simulink model "BLDCmotorControl_FOC_R2017b_fixdt_speedDeriv"  (R2017b)
settings: Solver=FixedStepDiscrete  StartTime=0  StopTime=0.5  FixedStep=Ts  MaxStep=1e-6  RelTol=1e-6  AbsTol=1e-6  EnableMultiTasking=on
PreLoadFcn:
  | addpath(genpath('01_Libraries'));
  | addpath(genpath('02_Figures'));
InitFcn:
  | init_model;
values from neighbouring files (symbols this model uses):
  a_elecAngle = 60    [init_model_Ffwd.m]
  b_DCLinkCurrAvail = 0    [init_model_Ffwd.m]
  b_fieldWeakEna = 0    [init_model_Ffwd.m]
  b_selPhaABCurrMeas = 1    [init_model_Ffwd.m]
  cf_currFilt = 0.02    [init_model_Ffwd.m]
  cf_speedCoef = round(f_ctrl * a_mechAngle * (pi/180) * (30/pi))    [init_model_Ffwd.m]
  CTRL_COM = 0    [init_model_Ffwd.m]
  dV_openRate = 1000 * Ts_ctrl    (= 0.06)    [init_model_Ffwd.m]
  dz_cntTrnsDetHi = 40    [init_model_Ffwd.m]
  dz_cntTrnsDetLo = 20    [init_model_Ffwd.m]
  i_max = i_max * i_sca    (= 750)    [init_model_Ffwd.m]
  i_thresOutlier = 200    [init_model_Ffwd.m]
  id_fieldWeak_M1 = [  0   0  0.05  0.25    1    2    3    4  4.5  4.8   5   5] * i_sca    [init_model_Ffwd.m]
  id_Kb = 1000 * Ts_ctrl    (= 0.06)    [init_model_Ffwd.m]
  id_Ki = 80 * Ts_ctrl    (= 0.0048)    [init_model_Ffwd.m]
  id_Kp = 0.5    [init_model_Ffwd.m]
  iq_Kb = 1000 * Ts_ctrl    (= 0.06)    [init_model_Ffwd.m]
  iq_Ki = 100 * Ts_ctrl    (= 0.006)    [init_model_Ffwd.m]
  iq_Kp = 0.5    [init_model_Ffwd.m]
  iq_KpLimProt = 4    [init_model_Ffwd.m]
  n_commAcvLo = 15    [init_model_Ffwd.m]
  n_commDeacvHi = 30    [init_model_Ffwd.m]
  n_Kb = 1000 * Ts_ctrl    (= 0.06)    [init_model_Ffwd.m]
  n_Ki = 10 * Ts_ctrl    (= 0.0006)    [init_model_Ffwd.m]
  n_Kp = 1    [init_model_Ffwd.m]
  n_KpLimProt = 5    [init_model_Ffwd.m]
  n_max = 800    [init_model_Ffwd.m]
  n_stdStillDet = 3    [init_model_Ffwd.m]
  OPEN_MODE = 0    [init_model_Ffwd.m]
  r_cos_M1 = cos((a_elecAngle_XA + 30)*(pi/180))    [init_model_Ffwd.m]
  r_sin_M1 = sin((a_elecAngle_XA + 30)*(pi/180))    [init_model_Ffwd.m]
  r_whl = 6.5 * 2.54 * 1e-2 / 2    (= 0.08255)    [init_model_Ffwd.m]
  SPD_MODE = 2    [init_model_Ffwd.m]
  TRQ_MODE = 3    [init_model_Ffwd.m]
  Ts = 5e-6    (= 5e-06)    [init_model_Ffwd.m]    (also in pe_electric_engine_dyno_data.m = 1e-05)
  Ts_ctrl = 6e-5    (= 6e-05)    [init_model_Ffwd.m]
  vec_hallToPos = [0 2 0 1 4 3 5 0]    [init_model_Ffwd.m]
  VLT_MODE = 1    [init_model_Ffwd.m]
  z_commutMap_M1 = [-1 -1  0  1  1  0 ... (first row only)    [init_model_Ffwd.m]
  z_ctrlModReq = 1    [init_model_Ffwd.m]
  z_ctrlTypSel = 1    [init_model_Ffwd.m]
  z_maxCntRst = 2000    [init_model_Ffwd.m]
undefined symbols (not defined in the file or in its folder): DiscIntNeverNeededParam, i_qMax_M1, sigbuilder_block, V_dMax, V_max, V_min, V_qMax_M1
libraries: simulink x11, BLDC_controller_Lib x9, powerlib x6, simulink_extras x1, pePwmGenerator x1
(part 2 of 3)

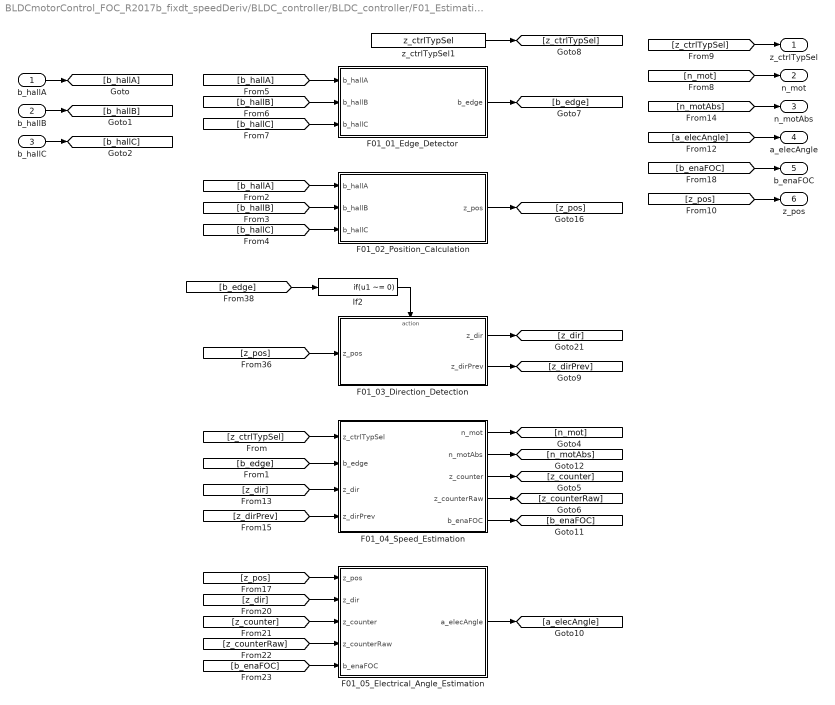
== system BLDCmotorControl_FOC_R2017b_fixdt_speedDeriv/BLDC_controller/BLDC_controller/F01_Estimations ==
  b_hallA : Inport
  b_hallB : Inport  Port=2
  b_hallC : Inport  Port=3
  F01_01_Edge_Detector : Subsystem
  F01_02_Position_Calculation : Subsystem
  F01_03_Direction_Detection : Subsystem
  F01_04_Speed_Estimation : Subsystem
  F01_05_Electrical_Angle_Estimation : Subsystem
  If2 : If  IfExpression=u1 ~= 0  ShowElse=off
  z_ctrlTypSel1 : Constant  Value=z_ctrlTypSel  OutDataTypeStr=uint8
  z_ctrlTypSel : Outport  OutputWhenDisabled=reset  InitialOutput=0
  "n_mot " : Outport  Port=2  OutputWhenDisabled=reset  InitialOutput=0
  n_motAbs : Outport  Port=3  OutputWhenDisabled=reset  InitialOutput=0
  a_elecAngle : Outport  Port=4  OutputWhenDisabled=reset  InitialOutput=0
  b_enaFOC : Outport  Port=5
  z_pos : Outport  Port=6  OutputWhenDisabled=reset  InitialOutput=0
  wires:
  If2/1 -> F01_03_Direction_Detection/Action
  [b_edge] -> If2/1
  [z_pos] -> F01_03_Direction_Detection/1(z_pos)
  [b_hallA] -> F01_01_Edge_Detector/1(b_hallA)
  F01_01_Edge_Detector/1("b_edge ") -> [b_edge]
  F01_03_Direction_Detection/1(z_dir) -> [z_dir]
  [b_hallB] -> F01_01_Edge_Detector/2(b_hallB)
  [b_hallC] -> F01_01_Edge_Detector/3(b_hallC)
  b_hallA/1 -> [b_hallA]
  b_hallB/1 -> [b_hallB]
  b_hallC/1 -> [b_hallC]
  [b_hallC] -> F01_02_Position_Calculation/3(b_hallC)
  [b_hallB] -> F01_02_Position_Calculation/2(b_hallB)
  [b_hallA] -> F01_02_Position_Calculation/1(b_hallA)
  F01_02_Position_Calculation/1("z_pos ") -> [z_pos]
  [b_edge] -> F01_04_Speed_Estimation/2(b_edge)
  F01_04_Speed_Estimation/1(n_mot) -> [n_mot]
  [n_mot] -> "n_mot "/1
  [z_pos] -> z_pos/1
  [z_dir] -> F01_04_Speed_Estimation/3(z_dir)
  F01_04_Speed_Estimation/3(z_counter) -> [z_counter]
  F01_04_Speed_Estimation/4(z_counterRaw) -> [z_counterRaw]
  F01_03_Direction_Detection/2(z_dirPrev) -> [z_dirPrev]
  [z_dirPrev] -> F01_04_Speed_Estimation/4(z_dirPrev)
  [z_pos] -> F01_05_Electrical_Angle_Estimation/1(z_pos)
  [z_dir] -> F01_05_Electrical_Angle_Estimation/2(z_dir)
  [z_counter] -> F01_05_Electrical_Angle_Estimation/3(z_counter)
  [z_counterRaw] -> F01_05_Electrical_Angle_Estimation/4(z_counterRaw)
  [b_enaFOC] -> F01_05_Electrical_Angle_Estimation/5(b_enaFOC)
  z_ctrlTypSel1/1 -> [z_ctrlTypSel]
  F01_04_Speed_Estimation/5(b_enaFOC) -> [b_enaFOC]
  [z_ctrlTypSel] -> F01_04_Speed_Estimation/1(z_ctrlTypSel)
  [b_enaFOC] -> b_enaFOC/1
  [a_elecAngle] -> a_elecAngle/1
  F01_05_Electrical_Angle_Estimation/1(a_elecAngle) -> [a_elecAngle]
  F01_04_Speed_Estimation/2(n_motAbs) -> [n_motAbs]
  [n_motAbs] -> n_motAbs/1
  [z_ctrlTypSel] -> z_ctrlTypSel/1

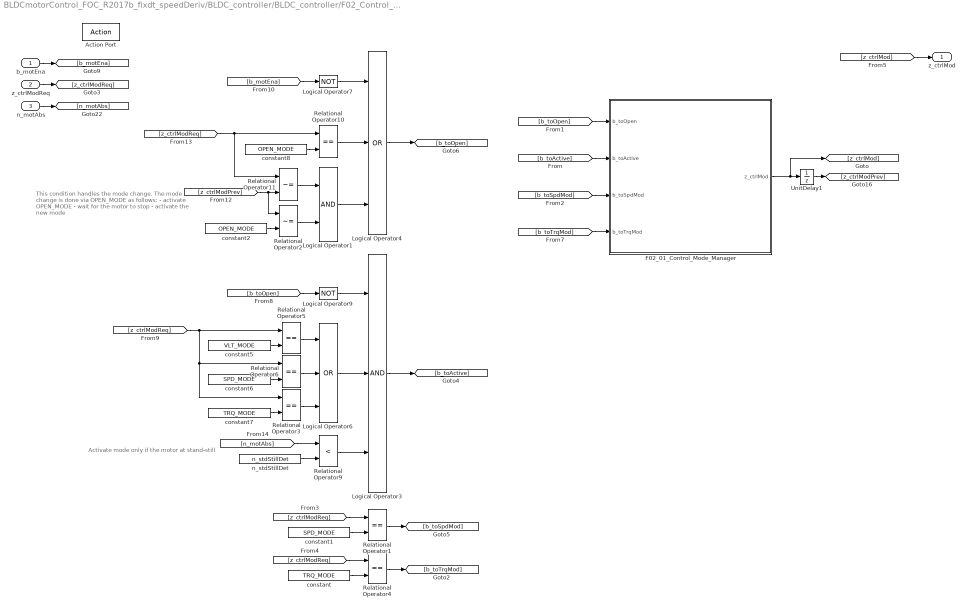
== system BLDCmotorControl_FOC_R2017b_fixdt_speedDeriv/BLDC_controller/BLDC_controller/F02_Control_Mode_Manager ==
  note: This condition handles the mode change. The mode change is done via OPEN_MODE as follows:
      | - activate OPEN_MODE
      | - wait for the motor to stop
      | - activate the new mode
  note: Activate mode only if the motor at stand-still
  b_motEna : Inport
  z_ctrlModReq : Inport  Port=2
  n_motAbs : Inport  Port=3
  Action Port : ActionPort  InitializeStates=reset  ActionType=then
  F02_01_Control_Mode_Manager : Stateflow chart  TreatAsAtomicUnit=on
  Logical Operator1 : Logic  AllPortsSameDT=off  OutDataTypeStr=boolean
  Logical Operator3 : Logic  Inputs=3  AllPortsSameDT=off  OutDataTypeStr=boolean
  Logical Operator4 : Logic  Operator=OR  Inputs=3  AllPortsSameDT=off  OutDataTypeStr=boolean
  Logical Operator6 : Logic  Operator=OR  Inputs=3  AllPortsSameDT=off  OutDataTypeStr=boolean
  Logical Operator7 : Logic  Operator=NOT  AllPortsSameDT=off  OutDataTypeStr=boolean
  Logical Operator9 : Logic  Operator=NOT  AllPortsSameDT=off  OutDataTypeStr=boolean
  Relational Operator{1,3..6,10} (6 alike) : RelationalOperator  Operator===  OutDataTypeStr=boolean  RndMeth=Simplest
  Relational Operator11 : RelationalOperator  Operator=~=  OutDataTypeStr=boolean  RndMeth=Simplest
  Relational Operator2 : RelationalOperator  Operator=~=  OutDataTypeStr=boolean  RndMeth=Simplest
  Relational Operator9 : RelationalOperator  Operator=<  OutDataTypeStr=boolean  RndMeth=Simplest
  UnitDelay1 : UnitDelay  SampleTime=-1
  constant : Constant  Value=TRQ_MODE  OutDataTypeStr=Inherit: Inherit via back propagation
  constant1 : Constant  Value=SPD_MODE  OutDataTypeStr=Inherit: Inherit via back propagation
  constant2 : Constant  Value=OPEN_MODE  OutDataTypeStr=Inherit: Inherit via back propagation
  constant5 : Constant  Value=VLT_MODE  OutDataTypeStr=Inherit: Inherit via back propagation
  constant6 : Constant  Value=SPD_MODE  OutDataTypeStr=Inherit: Inherit via back propagation
  constant7 : Constant  Value=TRQ_MODE  OutDataTypeStr=Inherit: Inherit via back propagation
  constant8 : Constant  Value=OPEN_MODE  OutDataTypeStr=Inherit: Inherit via back propagation
  n_stdStillDet : Constant  Value=n_stdStillDet  OutDataTypeStr=Inherit: Inherit via back propagation
  z_ctrlMod : Outport  OutputWhenDisabled=reset  InitialOutput=0
  wires:
  [z_ctrlMod] -> z_ctrlMod/1
  b_motEna/1 -> [b_motEna]
  [z_ctrlModReq] -> Relational Operator4/1
  constant/1 -> Relational Operator4/2
  Relational Operator4/1 -> [b_toTrqMod]
  [b_toOpen] -> F02_01_Control_Mode_Manager/1(b_toOpen)
  [b_toSpdMod] -> F02_01_Control_Mode_Manager/3(b_toSpdMod)
  z_ctrlModReq/1 -> [z_ctrlModReq]
  Relational Operator1/1 -> [b_toSpdMod]
  constant1/1 -> Relational Operator1/2
  [z_ctrlModReq] -> Relational Operator1/1
  [b_toTrqMod] -> F02_01_Control_Mode_Manager/4(b_toTrqMod)
  [z_ctrlModReq] -> Relational Operator6/1, Relational Operator3/1, Relational Operator5/1
  Relational Operator6/1 -> Logical Operator6/2
  constant6/1 -> Relational Operator6/2
  Relational Operator5/1 -> Logical Operator6/1
  constant5/1 -> Relational Operator5/2
  constant7/1 -> Relational Operator3/2
  Relational Operator3/1 -> Logical Operator6/3
  Logical Operator3/1 -> [b_toActive]
  [n_motAbs] -> Relational Operator9/1
  n_stdStillDet/1 -> Relational Operator9/2
  [z_ctrlModReq] -> Relational Operator11/1, Relational Operator10/1
  Logical Operator7/1 -> Logical Operator4/1
  [b_motEna] -> Logical Operator7/1
  Logical Operator4/1 -> [b_toOpen]
  [b_toOpen] -> Logical Operator9/1
  Logical Operator9/1 -> Logical Operator3/1
  UnitDelay1/1 -> [z_ctrlModPrev]
  F02_01_Control_Mode_Manager/1(z_ctrlMod) -> [z_ctrlMod], UnitDelay1/1
  [z_ctrlModPrev] -> Relational Operator2/1, Relational Operator11/2
  Relational Operator10/1 -> Logical Operator4/2
  constant8/1 -> Relational Operator10/2
  Logical Operator6/1 -> Logical Operator3/2
  Relational Operator9/1 -> Logical Operator3/3
  n_motAbs/1 -> [n_motAbs]
  [b_toActive] -> F02_01_Control_Mode_Manager/2(b_toActive)
  constant2/1 -> Relational Operator2/2
  Relational Operator11/1 -> Logical Operator1/1
  Relational Operator2/1 -> Logical Operator1/2
  Logical Operator1/1 -> Logical Operator4/3

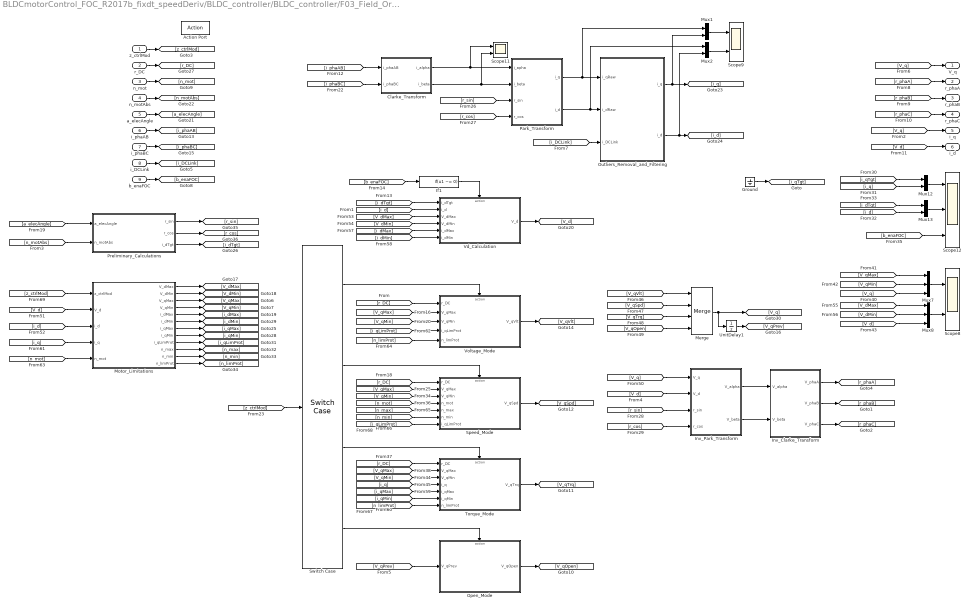
== system BLDCmotorControl_FOC_R2017b_fixdt_speedDeriv/BLDC_controller/BLDC_controller/F03_Field_Oriented_Control ==
  z_ctrlMod : Inport
  r_DC : Inport  Port=2
  n_mot : Inport  Port=3
  n_motAbs : Inport  Port=4
  a_elecAngle : Inport  Port=5
  i_phaAB : Inport  Port=6
  i_phaBC : Inport  Port=7
  i_DCLink : Inport  Port=8
  b_enaFOC : Inport  Port=9
  Action Port : ActionPort  InitializeStates=reset  ActionType=then
  Clarke_Transform : Subsystem
  Ground : Ground
  If1 : If  IfExpression=u1 ~= 0  ShowElse=off
  Inv_Clarke_Transform : Subsystem
  Inv_Park_Transform : Subsystem
  Merge : Merge  Inputs=4
  Motor_Limitations : Subsystem
  Mux{1..2,12..13} (4 alike) : Mux  Inputs=2
  Mux7 : Mux  Inputs=3
  Mux8 : Mux  Inputs=3
  Open_Mode : Subsystem
  Outliers_Removal_and_Filtering : Subsystem
  Park_Transform : Subsystem
  Preliminary_Calculations : Subsystem
  Scope11 : Scope  NumInputPorts=2
  Scope12 : Scope  NumInputPorts=3
  Scope8 : Scope  NumInputPorts=2
  Scope9 : Scope  NumInputPorts=2
  Speed_Mode : Subsystem
  Switch Case : SwitchCase  CaseConditions={VLT_MODE, SPD_MODE, TRQ_MODE}
  Torque_Mode : Subsystem
  UnitDelay1 : UnitDelay  SampleTime=-1
  Vd_Calculation : Subsystem
  Voltage_Mode : Subsystem
  V_q : Outport  OutputWhenDisabled=reset  InitialOutput=0
  r_phaA : Outport  Port=2  OutputWhenDisabled=reset  InitialOutput=0
  r_phaB : Outport  Port=3  OutputWhenDisabled=reset  InitialOutput=0
  "r_phaC " : Outport  Port=4  OutputWhenDisabled=reset  InitialOutput=0
  i_q : Outport  Port=5  OutputWhenDisabled=reset  InitialOutput=0
  i_d : Outport  Port=6  OutputWhenDisabled=reset  InitialOutput=0
  wires:
  [r_phaA] -> r_phaA/1
  [r_phaB] -> r_phaB/1
  [r_phaC] -> "r_phaC "/1
  Inv_Park_Transform/1(V_alpha) -> Inv_Clarke_Transform/1(V_alpha)
  Inv_Park_Transform/2(V_beta) -> Inv_Clarke_Transform/2(V_beta)
  i_phaAB/1 -> [i_phaAB]
  i_phaBC/1 -> [i_phaBC]
  Inv_Clarke_Transform/1(V_phaA) -> [r_phaA]
  Inv_Clarke_Transform/2(V_phaB) -> [r_phaB]
  Inv_Clarke_Transform/3(V_phaC) -> [r_phaC]
  Clarke_Transform/1(i_alpha) -> Scope11/1, Park_Transform/1(i_apha)
  Clarke_Transform/2(i_beta) -> Scope11/2, Park_Transform/2(i_beta)
  Mux12/1 -> Scope12/1
  Mux13/1 -> Scope12/2
  [r_sin] -> Park_Transform/3(r_sin)
  [r_cos] -> Park_Transform/4(r_cos)
  [r_sin] -> Inv_Park_Transform/3(r_sin)
  [r_cos] -> Inv_Park_Transform/4(r_cos)
  [i_qTgt] -> Mux12/1
  [i_q] -> Mux12/2
  [i_d] -> Mux13/2
  [i_dTgt] -> Mux13/1
  r_DC/1 -> [r_DC]
  [i_phaAB] -> Clarke_Transform/1(i_phaAB)
  [i_phaBC] -> Clarke_Transform/2(i_phaBC)
  [V_dMax] -> Mux8/1
  [V_d] -> Mux8/3
  Mux8/1 -> Scope8/2
  [V_dMin] -> Mux8/2
  [V_q] -> Mux7/3
  Mux7/1 -> Scope8/1
  [V_qMax] -> Mux7/1
  [V_qMin] -> Mux7/2
  [V_d] -> i_d/1
  [V_q] -> i_q/1
  [i_DCLink] -> Outliers_Removal_and_Filtering/3(i_DCLink)
  i_DCLink/1 -> [i_DCLink]
  Park_Transform/2(i_d) -> Mux2/1, Outliers_Removal_and_Filtering/2(i_dRaw)
  Park_Transform/1(i_q) -> Mux1/1, Outliers_Removal_and_Filtering/1(i_qRaw)
  Outliers_Removal_and_Filtering/1(i_q) -> Mux1/2, [i_q]
  Outliers_Removal_and_Filtering/2(i_d) -> Mux2/2, [i_d]
  [V_q] -> V_q/1
  Vd_Calculation/1(V_d) -> [V_d]
  [i_d] -> Vd_Calculation/2(i_d)
  [i_dTgt] -> Vd_Calculation/1(i_dTgt)
  b_enaFOC/1 -> [b_enaFOC]
  If1/1 -> Vd_Calculation/Action
  [b_enaFOC] -> If1/1
  [V_d] -> Inv_Park_Transform/2(V_d)
  z_ctrlMod/1 -> [z_ctrlMod]
  n_mot/1 -> [n_mot]
  [b_enaFOC] -> Scope12/3
  [z_ctrlMod] -> Switch Case/1
  [V_qPrev] -> Open_Mode/1(V_qPrev)
  Open_Mode/1(V_qOpen) -> [V_qOpen]
  Torque_Mode/1(V_qTrq) -> [V_qTrq]
  Speed_Mode/1(V_qSpd) -> [V_qSpd]
  Voltage_Mode/1(V_qVlt) -> [V_qVlt]
  [r_DC] -> Voltage_Mode/1(r_DC)
  [V_qMax] -> Voltage_Mode/2(V_qMax)
  [V_qMin] -> Voltage_Mode/3(V_qMin)
  [r_DC] -> Speed_Mode/1(r_DC)
  [V_qMax] -> Speed_Mode/2(V_qMax)
  [V_qMin] -> Speed_Mode/3(V_qMin)
  [n_mot] -> Speed_Mode/4(n_mot)
  [V_qMin] -> Torque_Mode/3(V_qMin)
  [V_qMax] -> Torque_Mode/2(V_qMax)
  [r_DC] -> Torque_Mode/1(r_DC)
  [i_q] -> Torque_Mode/4(i_q)
  Switch Case/1 -> Voltage_Mode/Action
  Switch Case/2 -> Speed_Mode/Action
  Switch Case/3 -> Torque_Mode/Action
  Switch Case/4 -> Open_Mode/Action
  [V_qVlt] -> Merge/1
  [V_qSpd] -> Merge/2
  [V_qTrq] -> Merge/3
  [V_qOpen] -> Merge/4
  [V_q] -> Inv_Park_Transform/1(V_q)
  Merge/1 -> UnitDelay1/1, [V_q]
  UnitDelay1/1 -> [V_qPrev]
  Motor_Limitations/3(V_qMax) -> [V_qMax]
  Motor_Limitations/4(V_qMin) -> [V_qMin]
  [V_d] -> Motor_Limitations/2(V_d)
  [i_d] -> Motor_Limitations/3(i_d)
  Motor_Limitations/2(V_dMin) -> [V_dMin]
  Motor_Limitations/1(V_dMax) -> [V_dMax]
  [V_dMax] -> Vd_Calculation/3(V_dMax)
  [V_dMin] -> Vd_Calculation/4(V_dMin)
  Motor_Limitations/5(i_dMax) -> [i_dMax]
  Motor_Limitations/6(i_dMin) -> [i_dMin]
  Motor_Limitations/7(i_qMax) -> [i_qMax]
  Motor_Limitations/8(i_qMin) -> [i_qMin]
  [i_dMax] -> Vd_Calculation/5(i_dMax)
  [i_dMin] -> Vd_Calculation/6(i_dMin)
  [i_qMax] -> Torque_Mode/5(i_qMax)
  [i_qMin] -> Torque_Mode/6(i_qMin)
  [i_q] -> Motor_Limitations/4(i_q)
  Motor_Limitations/9(i_qLimProt) -> [i_qLimProt]
  [i_qLimProt] -> Voltage_Mode/4(i_qLimProt)
  Motor_Limitations/11(n_min) -> [n_min]
  Motor_Limitations/10(n_max) -> [n_max]
  Motor_Limitations/12(n_limProt) -> [n_limProt]
  [n_mot] -> Motor_Limitations/5(n_mot)
  [n_limProt] -> Voltage_Mode/5(n_limProt)
  [n_max] -> Speed_Mode/5(n_max)
  [n_min] -> Speed_Mode/6(n_min)
  [n_limProt] -> Torque_Mode/7(n_limProt)
  [i_qLimProt] -> Speed_Mode/7(i_qLimProt)
  [z_ctrlMod] -> Motor_Limitations/1(z_ctrlMod)
  n_motAbs/1 -> [n_motAbs]
  Preliminary_Calculations/1(r_sin) -> [r_sin]
  Preliminary_Calculations/2(r_cos) -> [r_cos]
  [a_elecAngle] -> Preliminary_Calculations/1(a_elecAngle)
  Preliminary_Calculations/3(i_dTgt) -> [i_dTgt]
  [n_motAbs] -> Preliminary_Calculations/2(n_motAbs)
  a_elecAngle/1 -> [a_elecAngle]
  Ground/1 -> [i_qTgt]
  Mux1/1 -> Scope9/1
  Mux2/1 -> Scope9/2

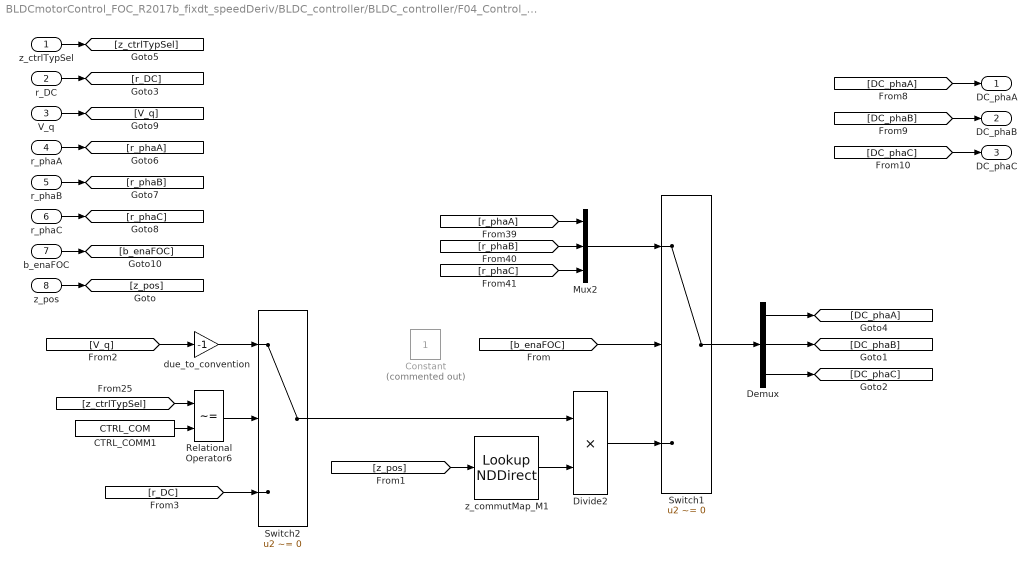
== system BLDCmotorControl_FOC_R2017b_fixdt_speedDeriv/BLDC_controller/BLDC_controller/F04_Control_Type_Management ==
  z_ctrlTypSel : Inport
  r_DC : Inport  Port=2
  V_q : Inport  Port=3
  r_phaA : Inport  Port=4
  r_phaB : Inport  Port=5
  r_phaC : Inport  Port=6
  b_enaFOC : Inport  Port=7
  z_pos : Inport  Port=8
  CTRL_COMM1 : Constant  Value=CTRL_COM  OutDataTypeStr=Inherit: Inherit via back propagation
  Constant : Constant  Commented=on  OutDataTypeStr=boolean
  Demux : Demux  Outputs=3
  Divide2 : Product  Inputs=**  RndMeth=Simplest  OutDataTypeStr=Inherit: Same as first input
  Mux2 : Mux  Inputs=3
  Relational Operator6 : RelationalOperator  Operator=~=  OutDataTypeStr=boolean  RndMeth=Simplest
  Switch1 : Switch  Criteria=u2 ~= 0  OutDataTypeStr=Inherit: Inherit via back propagation  RndMeth=Zero
  Switch2 : Switch  Criteria=u2 ~= 0  OutDataTypeStr=Inherit: Inherit via back propagation  RndMeth=Zero
  due_to_convention : Gain  Tag=struct('comment',struct('text','','placement',1),'logdata',struct('maxnumvals',inf,'plotchannels',[],'loggingmode',3,'channels',1),'output',struct('variable','','description','','name','$S_$B','width',1,'address','','max',NaN,'min',NaN,'class','default','type','CONTINUOUS','scaling','','lsb',1,'offset',0,'arb',0,'freeze',1,'unit','','autoscalingmode',1,'lowerheadroom',1,'upperheadroom',1,'headroomunit','bit','keepdatatype',1,'checkmin',0,'checkmax',0,'castoutput',0,'show',0),'gain',struct('variable','','description','','name','$S_$B_gain','width',1,'address','','max',NaN,'min',NaN,'class','default','type','CONTINUOUS','scaling','','lsb',1,'offset',0,'arb',0,'freeze',1,'unit','','keepdatatype',1,'value','1','scalar',0,'tolerance',1),'scalingvalid',0,'date',730486)  Gain=-1  RndMeth=Zero  SaturateOnIntegerOverflow=on  OutDataTypeStr=Inherit: Same as input  ParamDataTypeStr=Inherit: Same as input
  z_commutMap_M1 : LookupNDDirect  InputsSelectThisObjectFromTable=Column  Table=z_commutMap_M1  DiagnosticForOutOfRangeInput=None  TableDataTypeStr=int16
  DC_phaA : Outport  OutputWhenDisabled=reset  InitialOutput=0
  DC_phaB : Outport  Port=2  OutputWhenDisabled=reset  InitialOutput=0
  "DC_phaC " : Outport  Port=3  OutputWhenDisabled=reset  InitialOutput=0
  wires:
  Demux/3 -> [DC_phaC]
  Demux/2 -> [DC_phaB]
  Demux/1 -> [DC_phaA]
  z_pos/1 -> [z_pos]
  [DC_phaC] -> "DC_phaC "/1
  [DC_phaB] -> DC_phaB/1
  [DC_phaA] -> DC_phaA/1
  [z_pos] -> z_commutMap_M1/1
  Switch1/1 -> Demux/1
  r_phaA/1 -> [r_phaA]
  r_phaB/1 -> [r_phaB]
  r_phaC/1 -> [r_phaC]
  V_q/1 -> [V_q]
  [r_phaA] -> Mux2/1
  [r_phaB] -> Mux2/2
  [r_phaC] -> Mux2/3
  z_commutMap_M1/1 -> Divide2/2
  Divide2/1 -> Switch1/3
  b_enaFOC/1 -> [b_enaFOC]
  Mux2/1 -> Switch1/1
  [b_enaFOC] -> Switch1/2
  [V_q] -> due_to_convention/1
  Switch2/1 -> Divide2/1
  due_to_convention/1 -> Switch2/1
  [z_ctrlTypSel] -> Relational Operator6/1
  CTRL_COMM1/1 -> Relational Operator6/2
  Relational Operator6/1 -> Switch2/2
  r_DC/1 -> [r_DC]
  [r_DC] -> Switch2/3
  z_ctrlTypSel/1 -> [z_ctrlTypSel]

== system BLDCmotorControl_FOC_R2017b_fixdt_speedDeriv/BLDC_controller/BLDC_controller/Implemented_control_methods ==

== system BLDCmotorControl_FOC_R2017b_fixdt_speedDeriv/PWM_gates/PWM_generator1/__InputSSForSFun__ ==
  DC : Inport  SampleTime=Ts
  __UniqueOutportName__1__ : Outport
  wires:
  DC/1 -> __UniqueOutportName__1__/1

== system BLDCmotorControl_FOC_R2017b_fixdt_speedDeriv/PWM_gates/PWM_generator1/__OutputSSForSFun__ ==
  __UniqueInportName__1__ : Inport
  PWM : Outport
  wires:
  __UniqueInportName__1__/1 -> PWM/1

== system BLDCmotorControl_FOC_R2017b_fixdt_speedDeriv/PWM_gates/PWM_generator12/__InputSSForSFun__ ==
  DC : Inport  SampleTime=Ts
  __UniqueOutportName__1__ : Outport
  wires:
  DC/1 -> __UniqueOutportName__1__/1

== system BLDCmotorControl_FOC_R2017b_fixdt_speedDeriv/PWM_gates/PWM_generator12/__OutputSSForSFun__ ==
  __UniqueInportName__1__ : Inport
  PWM : Outport
  wires:
  __UniqueInportName__1__/1 -> PWM/1

== system BLDCmotorControl_FOC_R2017b_fixdt_speedDeriv/PWM_gates/PWM_generator2/__InputSSForSFun__ ==
  DC : Inport  SampleTime=Ts
  __UniqueOutportName__1__ : Outport
  wires:
  DC/1 -> __UniqueOutportName__1__/1

== system BLDCmotorControl_FOC_R2017b_fixdt_speedDeriv/PWM_gates/PWM_generator2/__OutputSSForSFun__ ==
  __UniqueInportName__1__ : Inport
  PWM : Outport
  wires:
  __UniqueInportName__1__/1 -> PWM/1

== system BLDCmotorControl_FOC_R2017b_fixdt_speedDeriv/PWM_gates/PWM_generator3/__InputSSForSFun__ ==
  DC : Inport  SampleTime=Ts
  __UniqueOutportName__1__ : Outport
  wires:
  DC/1 -> __UniqueOutportName__1__/1

== system BLDCmotorControl_FOC_R2017b_fixdt_speedDeriv/PWM_gates/PWM_generator3/__OutputSSForSFun__ ==
  __UniqueInportName__1__ : Inport
  PWM : Outport
  wires:
  __UniqueInportName__1__/1 -> PWM/1

== system BLDCmotorControl_FOC_R2017b_fixdt_speedDeriv/PWM_gates/PWM_generator4/__InputSSForSFun__ ==
  DC : Inport  SampleTime=Ts
  __UniqueOutportName__1__ : Outport
  wires:
  DC/1 -> __UniqueOutportName__1__/1

== system BLDCmotorControl_FOC_R2017b_fixdt_speedDeriv/PWM_gates/PWM_generator4/__OutputSSForSFun__ ==
  __UniqueInportName__1__ : Inport
  PWM : Outport
  wires:
  __UniqueInportName__1__/1 -> PWM/1

== system BLDCmotorControl_FOC_R2017b_fixdt_speedDeriv/PWM_gates/PWM_generator5/__InputSSForSFun__ ==
  DC : Inport  SampleTime=Ts
  __UniqueOutportName__1__ : Outport
  wires:
  DC/1 -> __UniqueOutportName__1__/1

== system BLDCmotorControl_FOC_R2017b_fixdt_speedDeriv/PWM_gates/PWM_generator5/__OutputSSForSFun__ ==
  __UniqueInportName__1__ : Inport
  PWM : Outport
  wires:
  __UniqueInportName__1__/1 -> PWM/1

== system BLDCmotorControl_FOC_R2017b_fixdt_speedDeriv/BLDC_controller/BLDC_controller/F01_Estimations/F01_01_Edge_Detector ==
  b_hallA : Inport
  b_hallB : Inport  Port=2
  b_hallC : Inport  Port=3
  Bitwise Operator : simulink/Logic and Bit Operations/Bitwise Operator  logicop=XOR  UseBitMask=off  NumInputPorts=6  BitMask=bin2dec('11011001')  BitMaskRealWorld=Stored Integer
  UnitDelay : UnitDelay  SampleTime=-1
  UnitDelay1 : UnitDelay  SampleTime=-1
  UnitDelay2 : UnitDelay  SampleTime=-1
  "b_edge " : Outport  OutputWhenDisabled=reset  InitialOutput=0
  wires:
  b_hallA/1 -> Bitwise Operator/1, UnitDelay/1
  b_hallC/1 -> Bitwise Operator/3, UnitDelay2/1
  b_hallB/1 -> Bitwise Operator/2, UnitDelay1/1
  Bitwise Operator/1 -> "b_edge "/1
  UnitDelay1/1 -> Bitwise Operator/5
  UnitDelay2/1 -> Bitwise Operator/6
  UnitDelay/1 -> Bitwise Operator/4

== system BLDCmotorControl_FOC_R2017b_fixdt_speedDeriv/BLDC_controller/BLDC_controller/F01_Estimations/F01_02_Position_Calculation ==
  note: This calculates the low resolution position based on Hall sensors.
  b_hallA : Inport
  b_hallB : Inport  Port=2
  b_hallC : Inport  Port=3
  Selector : Selector  IndexMode=Zero-based  InputPortWidth=length(vec_hallToPos)  IndexOptions=Index vector (port)  Indices=[1 3]  OutputSizes=1
  Sum : Sum  Inputs=+++  RndMeth=Simplest  OutDataTypeStr=Inherit: Same as first input
  g_Ha : Gain  Gain=4  OutDataTypeStr=Inherit: Inherit via back propagation  RndMeth=Zero  ParamDataTypeStr=Inherit: Same as input
  g_Hb : Gain  Gain=2  OutDataTypeStr=Inherit: Inherit via back propagation  RndMeth=Simplest  ParamDataTypeStr=Inherit: Same as input
  vec_hallToPos : Constant  Value=vec_hallToPos  OutDataTypeStr=int8
  "z_pos " : Outport  OutputWhenDisabled=reset  InitialOutput=0
  wires:
  b_hallC/1 -> Sum/3
  g_Ha/1 -> Sum/1
  g_Hb/1 -> Sum/2
  Sum/1 -> Selector/2
  b_hallA/1 -> g_Ha/1
  b_hallB/1 -> g_Hb/1
  vec_hallToPos/1 -> Selector/1
  Selector/1 -> "z_pos "/1

== system BLDCmotorControl_FOC_R2017b_fixdt_speedDeriv/BLDC_controller/BLDC_controller/F01_Estimations/F01_03_Direction_Detection ==
  z_pos : Inport
  Action Port : ActionPort  ActionType=then
  Constant20 : Constant  Value=-5  OutDataTypeStr=Inherit: Inherit via back propagation
  Constant23 : Constant  Value=-1  OutDataTypeStr=int8
  Constant24 : Constant  OutDataTypeStr=int8
  Constant8 : Constant  OutDataTypeStr=Inherit: Inherit via back propagation
  Logical Operator3 : Logic  Operator=OR  AllPortsSameDT=off  OutDataTypeStr=boolean
  Relational Operator1 : RelationalOperator  Operator===  OutDataTypeStr=boolean  RndMeth=Simplest
  Relational Operator6 : RelationalOperator  Operator===  OutDataTypeStr=boolean  RndMeth=Simplest
  Sum2 : Sum  Inputs=|+-  RndMeth=Zero  InputSameDT=on  OutDataTypeStr=Inherit: Same as first input
  Switch2 : Switch  Criteria=u2 ~= 0  OutDataTypeStr=Inherit: Inherit via back propagation  RndMeth=Simplest
  UnitDelay1 : UnitDelay  SampleTime=-1
  UnitDelay2 : UnitDelay  SampleTime=-1
  z_dir : Outport
  z_dirPrev : Outport  Port=2
  wires:
  UnitDelay2/1 -> Sum2/2
  Relational Operator1/1 -> Logical Operator3/1
  Constant8/1 -> Relational Operator1/2
  Sum2/1 -> Relational Operator6/1, Relational Operator1/1
  Relational Operator6/1 -> Logical Operator3/2
  Constant20/1 -> Relational Operator6/2
  Constant24/1 -> Switch2/1
  Constant23/1 -> Switch2/3
  Logical Operator3/1 -> Switch2/2
  z_pos/1 -> Sum2/1, UnitDelay2/1
  Switch2/1 -> UnitDelay1/1, z_dir/1
  UnitDelay1/1 -> z_dirPrev/1

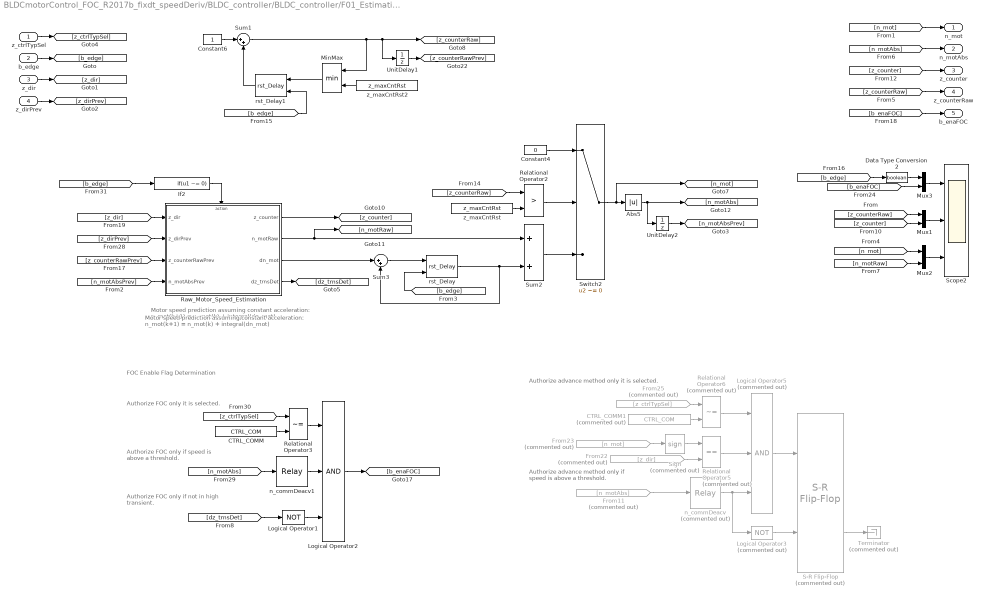
== system BLDCmotorControl_FOC_R2017b_fixdt_speedDeriv/BLDC_controller/BLDC_controller/F01_Estimations/F01_04_Speed_Estimation ==
  note: Motor speed prediction assuming constant acceleration:
      | n_mot(k+1) = n_mot(k) + integral(dn_mot)
  note: Authorize advance method only if speed is above a threshold.
  note: Authorize advance method only it is selected.
  note: FOC Enable Flag Determination
  note: Authorize FOC only if speed is above a threshold.
  note: Authorize FOC only if not in high transient.
  note: Authorize FOC only it is selected.
  note: Motor speed prediction assuming constant acceleration:
      | n_mot(k+1) = n_mot(k) + integral(dn_mot)
  z_ctrlTypSel : Inport
  b_edge : Inport  Port=2
  z_dir : Inport  Port=3
  z_dirPrev : Inport  Port=4
  Abs5 : Abs  OutDataTypeStr=Inherit: Inherit via back propagation  RndMeth=Zero
  CTRL_COMM : Constant  Value=CTRL_COM  OutDataTypeStr=Inherit: Inherit via back propagation
  CTRL_COMM1 : Constant  Commented=on  Value=CTRL_COM  OutDataTypeStr=Inherit: Inherit via back propagation
  Constant4 : Constant  Value=0  OutDataTypeStr=Inherit: Inherit via back propagation
  Constant6 : Constant  OutDataTypeStr=int16
  Data Type Conversion2 : DataTypeConversion  OutDataTypeStr=boolean
  From11 : From  Commented=on  GotoTag=n_motAbs
  From22 : From  Commented=on  GotoTag=z_dir
  From23 : From  Commented=on  GotoTag=n_mot
  From25 : From  Commented=on  GotoTag=z_ctrlTypSel
  If2 : If  IfExpression=u1 ~= 0  ShowElse=off
  Logical Operator1 : Logic  Operator=NOT  AllPortsSameDT=off  OutDataTypeStr=boolean
  Logical Operator2 : Logic  Inputs=3  AllPortsSameDT=off  OutDataTypeStr=boolean
  Logical Operator3 : Logic  Commented=on  Operator=NOT  AllPortsSameDT=off  OutDataTypeStr=boolean
  Logical Operator5 : Logic  Commented=on  Inputs=3  AllPortsSameDT=off  OutDataTypeStr=boolean
  MinMax : MinMax  Inputs=2
  Mux1 : Mux  Inputs=2
  Mux2 : Mux  Inputs=2
  Mux3 : Mux  Inputs=2
  Raw_Motor_Speed_Estimation : Subsystem
  Relational Operator2 : RelationalOperator  Operator=>  OutDataTypeStr=boolean  RndMeth=Simplest
  Relational Operator3 : RelationalOperator  Operator=~=  OutDataTypeStr=boolean  RndMeth=Simplest
  Relational Operator5 : RelationalOperator  Commented=on  Operator===  OutDataTypeStr=boolean  RndMeth=Simplest
  Relational Operator6 : RelationalOperator  Commented=on  Operator=~=  OutDataTypeStr=boolean  RndMeth=Simplest
  S-R Flip-Flop : simulink_extras/Flip Flops/S-R Flip-Flop  Commented=on  initial_condition=0
  Scope2 : Scope  NumInputPorts=3
  Sign : Signum  Commented=on
  Sum1 : Sum  Inputs=|++  RndMeth=Simplest  InputSameDT=on  OutDataTypeStr=Inherit: Same as first input
  Sum2 : Sum  RndMeth=Simplest  OutDataTypeStr=Inherit: Same as first input
  Sum3 : Sum  Inputs=|++  RndMeth=Simplest  OutDataTypeStr=Inherit: Same as first input
  Switch2 : Switch  Criteria=u2 ~= 0  OutDataTypeStr=Inherit: Inherit via back propagation  RndMeth=Zero
  Terminator : Terminator  Commented=on
  UnitDelay1 : UnitDelay  InitialCondition=z_maxCntRst  SampleTime=-1
  UnitDelay2 : UnitDelay  SampleTime=-1
  n_commDeacv : Relay  Commented=on  OnSwitchValue=n_commDeacvHi  OffSwitchValue=n_commAcvLo  OutDataTypeStr=boolean
  n_commDeacv1 : Relay  OnSwitchValue=n_commDeacvHi  OffSwitchValue=n_commAcvLo  OutDataTypeStr=boolean
  rst_Delay : BLDC_controller_Lib/rst_Delay  initVal=0
  rst_Delay1 : BLDC_controller_Lib/rst_Delay  initVal=z_maxCntRst
  z_maxCntRst : Constant  Value=z_maxCntRst  OutDataTypeStr=Inherit: Inherit via back propagation
  z_maxCntRst2 : Constant  Value=z_maxCntRst  OutDataTypeStr=Inherit: Inherit via back propagation
  n_mot : Outport
  n_motAbs : Outport  Port=2
  z_counter : Outport  Port=3  OutputWhenDisabled=reset  InitialOutput=0
  z_counterRaw : Outport  Port=4  OutputWhenDisabled=reset  InitialOutput=0
  b_enaFOC : Outport  Port=5
  wires:
  [n_motRaw] -> Mux2/2
  Mux2/1 -> Scope2/3
  [n_mot] -> Mux2/1
  Mux1/1 -> Scope2/2
  [z_counterRaw] -> Mux1/1
  [z_counter] -> Mux1/2
  [b_edge] -> Data Type Conversion2/1
  Constant6/1 -> Sum1/1
  Sum1/1 -> MinMax/1, [z_counterRaw], UnitDelay1/1
  b_edge/1 -> [b_edge]
  [n_mot] -> n_mot/1
  z_dir/1 -> [z_dir]
  [z_counter] -> z_counter/1
  [z_counterRaw] -> z_counterRaw/1
  UnitDelay1/1 -> [z_counterRawPrev]
  z_dirPrev/1 -> [z_dirPrev]
  Raw_Motor_Speed_Estimation/2(n_motRaw) -> Sum2/1, [n_motRaw]
  Raw_Motor_Speed_Estimation/3(dn_mot) -> Sum3/1
  [z_dir] -> Raw_Motor_Speed_Estimation/1(z_dir)
  Abs5/1 -> UnitDelay2/1, [n_motAbs]
  Raw_Motor_Speed_Estimation/1(z_counter) -> [z_counter]
  [z_dirPrev] -> Raw_Motor_Speed_Estimation/2(z_dirPrev)
  If2/1 -> Raw_Motor_Speed_Estimation/Action
  [z_counterRawPrev] -> Raw_Motor_Speed_Estimation/3(z_counterRawPrev)
  [b_enaFOC] -> b_enaFOC/1
  z_ctrlTypSel/1 -> [z_ctrlTypSel]
  rst_Delay/1 -> Sum2/2, Sum3/2
  [z_counterRaw] -> Relational Operator2/1
  z_maxCntRst/1 -> Relational Operator2/2
  Constant4/1 -> Switch2/1
  Sum2/1 -> Switch2/3
  Switch2/1 -> [n_mot], Abs5/1
  [b_edge] -> rst_Delay1/2
  z_maxCntRst2/1 -> MinMax/2
  rst_Delay1/1 -> Sum1/2
  MinMax/1 -> rst_Delay1/1
  S-R Flip-Flop/2 -> Terminator/1
  From11/1 -> n_commDeacv/1
  Logical Operator3/1 -> S-R Flip-Flop/2
  n_commDeacv/1 -> Logical Operator3/1, Logical Operator5/3
  Logical Operator5/1 -> S-R Flip-Flop/1
  Sign/1 -> Relational Operator5/1
  Relational Operator5/1 -> Logical Operator5/2
  Mux3/1 -> Scope2/1
  [b_enaFOC] -> Mux3/2
  Data Type Conversion2/1 -> Mux3/1
  From22/1 -> Relational Operator5/2
  From23/1 -> Sign/1
  From25/1 -> Relational Operator6/1
  CTRL_COMM1/1 -> Relational Operator6/2
  Relational Operator6/1 -> Logical Operator5/1
  [b_edge] -> If2/1
  Relational Operator2/1 -> Switch2/2
  UnitDelay2/1 -> [n_motAbsPrev]
  [n_motAbsPrev] -> Raw_Motor_Speed_Estimation/4(n_motAbsPrev)
  Sum3/1 -> rst_Delay/1
  [b_edge] -> rst_Delay/2
  [n_motAbs] -> n_motAbs/1
  CTRL_COMM/1 -> Relational Operator3/2
  [z_ctrlTypSel] -> Relational Operator3/1
  [n_motAbs] -> n_commDeacv1/1
  Raw_Motor_Speed_Estimation/4(dz_trnsDet) -> [dz_trnsDet]
  Relational Operator3/1 -> Logical Operator2/1
  n_commDeacv1/1 -> Logical Operator2/2
  Logical Operator1/1 -> Logical Operator2/3
  Logical Operator2/1 -> [b_enaFOC]
  [dz_trnsDet] -> Logical Operator1/1

== system BLDCmotorControl_FOC_R2017b_fixdt_speedDeriv/BLDC_controller/BLDC_controller/F01_Estimations/F01_05_Electrical_Angle_Estimation ==
  note: Electrical angle calculation
  note: This switch is to manage the situation when FOC control method is not enabled.
  z_pos : Inport
  z_dir : Inport  Port=2
  z_counter : Inport  Port=3
  z_counterRaw : Inport  Port=4
  b_enaFOC : Inport  Port=5
  Constant16 : Constant  OutDataTypeStr=Inherit: Inherit via back propagation
  Constant2 : Constant  OutDataTypeStr=Inherit: Inherit via back propagation
  Divide4 : Product  Inputs=*/*  RndMeth=Simplest  SaturateOnIntegerOverflow=on  OutDataTypeStr=Inherit: Same as first input
  Divide5 : Product  Inputs=**  RndMeth=Simplest  OutDataTypeStr=Inherit: Same as first input
  Mux : Mux  Inputs=2
  Product6 : Product  OutDataTypeStr=Inherit: Inherit via back propagation  RndMeth=Simplest
  Relational Operator7 : RelationalOperator  Operator===  OutDataTypeStr=boolean  RndMeth=Simplest
  Scope : Scope  NumInputPorts=2
  Sum1 : Sum  RndMeth=Simplest  OutDataTypeStr=Inherit: Same as first input
  Sum2 : Sum  RndMeth=Simplest  OutDataTypeStr=Inherit: Same as first input
  Switch1 : Switch  Criteria=u2 ~= 0  OutDataTypeStr=Inherit: Inherit via back propagation  RndMeth=Zero
  Switch3 : Switch  Criteria=u2 ~= 0  OutDataTypeStr=Inherit: Inherit via back propagation  RndMeth=Zero
  a_elecAngle1 : Constant  Value=a_elecAngle  OutDataTypeStr=fixdt(1,16,6)
  a_elecAngle : Outport  OutputWhenDisabled=reset  InitialOutput=0
  wires:
  z_pos/1 -> [z_pos]
  z_dir/1 -> [z_dir]
  Mux/1 -> Scope/1
  [a_elecAngle] -> Mux/1
  [a_elecAngleLowRes] -> Mux/2
  [b_enaFOC] -> Scope/2
  z_counterRaw/1 -> [z_counterRaw]
  z_counter/1 -> [z_counter]
  [z_counter] -> Divide4/2
  Switch3/1 -> Divide5/2
  [z_pos] -> Switch3/1, Sum1/1
  Constant2/1 -> Sum1/2
  Product6/1 -> Sum2/2
  Relational Operator7/1 -> Switch3/2
  Constant16/1 -> Relational Operator7/2
  a_elecAngle1/1 -> Divide5/1, Divide4/1
  [z_dir] -> Relational Operator7/1
  Sum1/1 -> Switch3/3
  Divide4/1 -> Product6/1
  Divide5/1 -> [a_elecAngleLowRes], Sum2/1
  b_enaFOC/1 -> [b_enaFOC]
  [b_enaFOC] -> Switch1/2
  Switch1/1 -> [a_elecAngle]
  Sum2/1 -> [a_elecAngleRaw]
  [a_elecAngleRaw] -> Switch1/1
  [a_elecAngleLowRes] -> Switch1/3
  [z_dir] -> Product6/2
  [z_counterRaw] -> Divide4/3
  [a_elecAngle] -> a_elecAngle/1

== system BLDCmotorControl_FOC_R2017b_fixdt_speedDeriv/BLDC_controller/BLDC_controller/F03_Field_Oriented_Control/Clarke_Transform ==
  i_phaAB : Inport
  i_phaBC : Inport  Port=2
  Clarke_PhasesAB : Subsystem
  Clarke_PhasesBC : Subsystem
  If1 : If  IfExpression=u1 ~= 0
  Merge : Merge
  Merge1 : Merge
  b_selPhaABCurrMeas : Constant  Value=b_selPhaABCurrMeas  OutDataTypeStr=boolean
  i_alpha : Outport
  i_beta : Outport  Port=2
  wires:
  Clarke_PhasesBC/1(i_alphaBC) -> [i_alphaBC]
  [i_betaBC] -> Merge1/2
  [i_betaAB] -> Merge1/1
  i_phaAB/1 -> [i_phaAB]
  [i_phaBC] -> Clarke_PhasesBC/2(i_phaC)
  [i_phaAB] -> Clarke_PhasesBC/1(i_phaB)
  Clarke_PhasesAB/1(i_alphaAB) -> [i_alphaAB]
  [i_alphaAB] -> Merge/1
  If1/1 -> Clarke_PhasesAB/Action
  b_selPhaABCurrMeas/1 -> If1/1
  If1/2 -> Clarke_PhasesBC/Action
  [i_alphaBC] -> Merge/2
  [i_beta] -> i_beta/1
  Clarke_PhasesAB/2(i_betaAB) -> [i_betaAB]
  i_phaBC/1 -> [i_phaBC]
  [i_phaBC] -> Clarke_PhasesAB/2(i_phaB)
  Merge1/1 -> [i_beta]
  Merge/1 -> [i_alpha]
  [i_phaAB] -> Clarke_PhasesAB/1(i_phaA)
  [i_alpha] -> i_alpha/1
  Clarke_PhasesBC/2(i_betaBC) -> [i_betaBC]

== system BLDCmotorControl_FOC_R2017b_fixdt_speedDeriv/BLDC_controller/BLDC_controller/F03_Field_Oriented_Control/Inv_Clarke_Transform ==
  note: Inverse Clarke Transform:
      | V_phaA = V_alpha
      | V_phaB = -(1/2)*V_alpha + (sqrt(3)/2)*V_beta
      | V_phaC = -VphaA - V_phaB
  note: Space Vector Modulation (SVM)
  V_alpha : Inport
  V_beta : Inport  Port=2
  Add : Sum
  Add1 : Sum  Inputs=-+
  Demux : Demux  Outputs=3
  Gain1 : Gain  Tag=struct('comment',struct('text','','placement',1),'logdata',struct('maxnumvals',inf,'plotchannels',[],'loggingmode',3,'channels',1),'output',struct('variable','','description','','name','$S_$B','width',1,'address','','max',NaN,'min',NaN,'class','default','type','CONTINUOUS','scaling','','lsb',1,'offset',0,'arb',0,'freeze',1,'unit','','autoscalingmode',1,'lowerheadroom',1,'upperheadroom',1,'headroomunit','bit','keepdatatype',1,'checkmin',0,'checkmax',0,'castoutput',0,'show',0),'gain',struct('variable','','description','','name','$S_$B_gain','width',1,'address','','max',NaN,'min',NaN,'class','default','type','CONTINUOUS','scaling','','lsb',1,'offset',0,'arb',0,'freeze',1,'unit','','keepdatatype',1,'value','1','scalar',0,'tolerance',1),'scalingvalid',0,'date',730486)  Gain=sqrt(3)/2  RndMeth=Zero
  Gain2 : Gain  Gain=0.5
  Gain3 : Gain  Tag=struct('comment',struct('text','','placement',1),'logdata',struct('maxnumvals',inf,'plotchannels',[],'loggingmode',3,'channels',1),'output',struct('variable','','description','','name','$S_$B','width',1,'address','','max',NaN,'min',NaN,'class','default','type','CONTINUOUS','scaling','','lsb',1,'offset',0,'arb',0,'freeze',1,'unit','','autoscalingmode',1,'lowerheadroom',1,'upperheadroom',1,'headroomunit','bit','keepdatatype',1,'checkmin',0,'checkmax',0,'castoutput',0,'show',0),'gain',struct('variable','','description','','name','$S_$B_gain','width',1,'address','','max',NaN,'min',NaN,'class','default','type','CONTINUOUS','scaling','','lsb',1,'offset',0,'arb',0,'freeze',1,'unit','','keepdatatype',1,'value','1','scalar',0,'tolerance',1),'scalingvalid',0,'date',730486)  Gain=1/2  RndMeth=Zero
  Gain4 : Gain  Gain=2/sqrt(3)  OutDataTypeStr=fixdt(1,16,0)
  MinMax1 : MinMax  InputSameDT=on
  MinMax2 : MinMax  Function=max  InputSameDT=on
  Mux4 : Mux  Inputs=3
  Sum2 : Sum  Inputs=--  OutDataTypeStr=fixdt(1,16,4)  RndMeth=Simplest
  Sum6 : Sum  Inputs=-+  OutDataTypeStr=fixdt(1,16,4)  RndMeth=Simplest
  V_phaA : Outport
  V_phaB : Outport  Port=2
  V_phaC : Outport  Port=3
  wires:
  Sum6/1 -> Sum2/2, Mux4/2
  Sum2/1 -> Mux4/3
  Gain1/1 -> Sum6/2
  Gain3/1 -> Sum6/1
  V_alpha/1 -> Gain3/1, Sum2/1, Mux4/1  "alpha"
  V_beta/1 -> Gain1/1  "beta"
  Add/1 -> Gain2/1
  Add1/1 -> Gain4/1
  MinMax1/1 -> Add/1
  Demux/3 -> V_phaC/1
  Demux/2 -> V_phaB/1
  Gain2/1 -> Add1/1
  Demux/1 -> V_phaA/1
  MinMax2/1 -> Add/2
  Mux4/1 -> Add1/2, MinMax2/1, MinMax1/1
  Gain4/1 -> Demux/1

== system BLDCmotorControl_FOC_R2017b_fixdt_speedDeriv/BLDC_controller/BLDC_controller/F03_Field_Oriented_Control/Inv_Park_Transform ==
  note: Inverse Park Transform:
      | V_alpha = V_d*cos(angle) - V_q*sin(angle)
      | V_beta = V_d*sin(angle) + V_q*cos(angle)
  V_q : Inport
  V_d : Inport  Port=2
  r_sin : Inport  Port=3
  r_cos : Inport  Port=4
  Divide{1..4} (4 alike) : Product  Inputs=**  RndMeth=Simplest
  Sum1 : Sum  OutDataTypeStr=fixdt(1,16,4)  RndMeth=Simplest
  Sum6 : Sum  Inputs=+-  OutDataTypeStr=fixdt(1,16,4)  RndMeth=Simplest
  V_alpha : Outport
  V_beta : Outport  Port=2
  wires:
  r_sin/1 -> [r_sin]
  V_d/1 -> [V_d]
  V_q/1 -> [V_q]
  r_cos/1 -> [r_cos]
  [r_cos] -> Divide4/2
  [r_sin] -> Divide1/2
  [V_d] -> Divide4/1
  [r_cos] -> Divide3/2
  Divide1/1 -> Sum6/2
  [V_q] -> Divide1/1
  [V_d] -> Divide2/1
  Divide2/1 -> Sum1/1
  Divide3/1 -> Sum1/2
  [V_q] -> Divide3/1
  Divide4/1 -> Sum6/1
  [r_sin] -> Divide2/2
  Sum1/1 -> V_beta/1
  Sum6/1 -> V_alpha/1

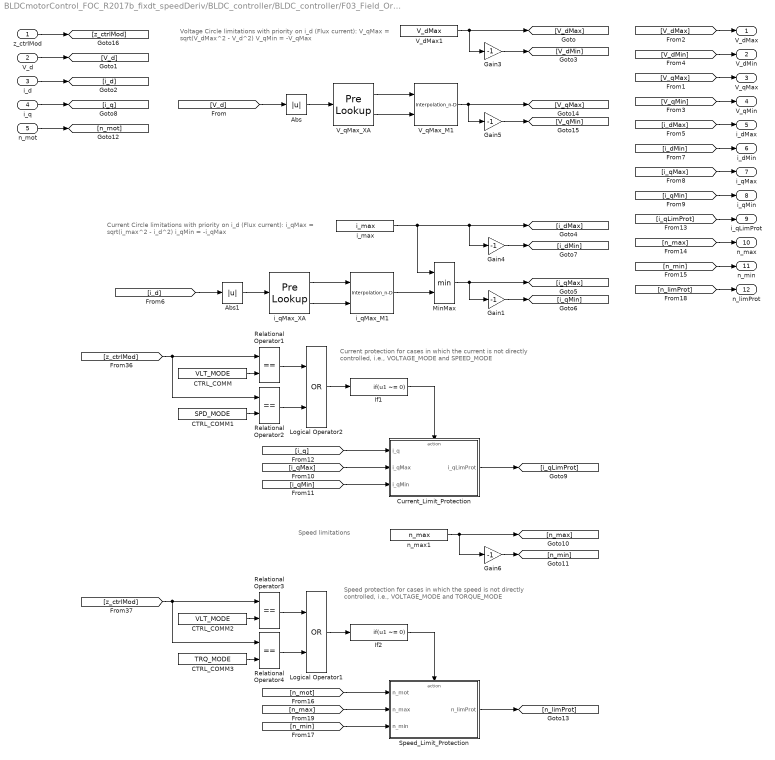
== system BLDCmotorControl_FOC_R2017b_fixdt_speedDeriv/BLDC_controller/BLDC_controller/F03_Field_Oriented_Control/Motor_Limitations ==
  note: Voltage Circle limitations with priority on i_d (Flux current):
      | V_qMax = sqrt(V_dMax^2 - V_d^2)
      | V_qMin = -V_qMax
  note: Current Circle limitations with priority on i_d (Flux current):
      | i_qMax = sqrt(i_max^2 - i_d^2)
      | i_qMin = -i_qMax
  note: Speed limitations
  note: Current protection
      | for cases in which the current is not directly controlled, i.e., VOLTAGE_MODE and SPEED_MODE
  note: Speed protection
      | for cases in which the speed is not directly controlled, i.e., VOLTAGE_MODE and TORQUE_MODE
  z_ctrlMod : Inport
  V_d : Inport  Port=2
  i_d : Inport  Port=3
  i_q : Inport  Port=4
  n_mot : Inport  Port=5
  Abs : Abs
  Abs1 : Abs
  CTRL_COMM : Constant  Value=VLT_MODE  OutDataTypeStr=Inherit: Inherit via back propagation
  CTRL_COMM1 : Constant  Value=SPD_MODE  OutDataTypeStr=Inherit: Inherit via back propagation
  CTRL_COMM2 : Constant  Value=VLT_MODE  OutDataTypeStr=Inherit: Inherit via back propagation
  CTRL_COMM3 : Constant  Value=TRQ_MODE  OutDataTypeStr=Inherit: Inherit via back propagation
  Current_Limit_Protection : Subsystem
  Gain{1,3..6} (5 alike) : Gain  Tag=struct('comment',struct('text','','placement',1),'logdata',struct('maxnumvals',inf,'plotchannels',[],'loggingmode',3,'channels',1),'output',struct('variable','','description','','name','$S_$B','width',1,'address','','max',NaN,'min',NaN,'class','default','type','CONTINUOUS','scaling','','lsb',1,'offset',0,'arb',0,'freeze',1,'unit','','autoscalingmode',1,'lowerheadroom',1,'upperheadroom',1,'headroomunit','bit','keepdatatype',1,'checkmin',0,'checkmax',0,'castoutput',0,'show',0),'gain',struct('variable','','description','','name','$S_$B_gain','width',1,'address','','max',NaN,'min',NaN,'class','default','type','CONTINUOUS','scaling','','lsb',1,'offset',0,'arb',0,'freeze',1,'unit','','keepdatatype',1,'value','1','scalar',0,'tolerance',1),'scalingvalid',0,'date',730486)  Gain=-1  RndMeth=Zero  OutDataTypeStr=Inherit: Same as input  ParamDataTypeStr=Inherit: Same as input
  If1 : If  IfExpression=u1 ~= 0  ShowElse=off
  If2 : If  IfExpression=u1 ~= 0  ShowElse=off
  Logical Operator1 : Logic  Operator=OR  AllPortsSameDT=off  OutDataTypeStr=boolean
  Logical Operator2 : Logic  Operator=OR  AllPortsSameDT=off  OutDataTypeStr=boolean
  MinMax : MinMax  Inputs=2
  Relational Operator{1..4} (4 alike) : RelationalOperator  Operator===  OutDataTypeStr=boolean  RndMeth=Simplest
  Speed_Limit_Protection : Subsystem
  V_dMax1 : Constant  Value=V_dMax  OutDataTypeStr=fixdt(1,16,4)
  V_qMax_M1 : Interpolation_n-D  NumberOfTableDimensions=1  Table=V_qMax_M1  ExtrapMethod=Clip  OutDataTypeStr=fixdt(1,16,4)  InternalRulePriority=Speed  RndMeth=Simplest
      settings: InputPortMap=u0,u1
  V_qMax_XA : PreLookup  BreakpointsData=V_qMax_XA  IndexSearchMethod=Evenly spaced points  BeginIndexSearchUsingPreviousIndexResult=on  IndexDataTypeStr=uint8  FractionDataTypeStr=fixdt(0,16,14)  RndMeth=Simplest
  i_max : Constant  Value=i_max  OutDataTypeStr=fixdt(1,16,4)
  i_qMax_M1 : Interpolation_n-D  NumberOfTableDimensions=1  Table=i_qMax_M1  ExtrapMethod=Clip  OutDataTypeStr=fixdt(1,16,4)  InternalRulePriority=Speed  RndMeth=Simplest
      settings: InputPortMap=u0,u1
  i_qMax_XA : PreLookup  BreakpointsData=i_qMax_XA  IndexSearchMethod=Evenly spaced points  BeginIndexSearchUsingPreviousIndexResult=on  IndexDataTypeStr=uint8  FractionDataTypeStr=fixdt(0,16,14)  RndMeth=Simplest
  n_max1 : Constant  Value=n_max  OutDataTypeStr=fixdt(1,16,4)
  V_dMax : Outport  OutputWhenDisabled=reset  InitialOutput=V_max
  V_dMin : Outport  Port=2  OutputWhenDisabled=reset  InitialOutput=V_min
  V_qMax : Outport  Port=3  OutputWhenDisabled=reset  InitialOutput=V_max
  V_qMin : Outport  Port=4  OutputWhenDisabled=reset  InitialOutput=V_min
  i_dMax : Outport  Port=5  OutputWhenDisabled=reset  InitialOutput=V_max
  i_dMin : Outport  Port=6  OutputWhenDisabled=reset  InitialOutput=V_min
  i_qMax : Outport  Port=7  OutputWhenDisabled=reset  InitialOutput=V_max
  i_qMin : Outport  Port=8  OutputWhenDisabled=reset  InitialOutput=V_min
  i_qLimProt : Outport  Port=9  OutputWhenDisabled=reset  InitialOutput=V_min
  n_max : Outport  Port=10  OutputWhenDisabled=reset  InitialOutput=V_max
  n_min : Outport  Port=11  OutputWhenDisabled=reset  InitialOutput=V_min
  n_limProt : Outport  Port=12  OutputWhenDisabled=reset  InitialOutput=V_min
  wires:
  V_qMax_XA/1 -> V_qMax_M1/1
  V_qMax_XA/2 -> V_qMax_M1/2
  [V_qMin] -> V_qMin/1
  [V_qMax] -> V_qMax/1
  Gain5/1 -> [V_qMin]
  V_qMax_M1/1 -> [V_qMax], Gain5/1
  Abs/1 -> V_qMax_XA/1
  V_d/1 -> [V_d]
  [V_d] -> Abs/1
  i_d/1 -> [i_d]
  [V_dMax] -> V_dMax/1
  [V_dMin] -> V_dMin/1
  V_dMax1/1 -> Gain3/1, [V_dMax]
  Gain3/1 -> [V_dMin]
  Gain4/1 -> [i_dMin]
  i_max/1 -> MinMax/1, Gain4/1, [i_dMax]
  [i_d] -> Abs1/1
  Abs1/1 -> i_qMax_XA/1
  MinMax/1 -> [i_qMax], Gain1/1
  Gain1/1 -> [i_qMin]
  i_qMax_XA/2 -> i_qMax_M1/2
  i_qMax_XA/1 -> i_qMax_M1/1
  [i_dMin] -> i_dMin/1
  [i_dMax] -> i_dMax/1
  [i_qMax] -> i_qMax/1
  [i_qMin] -> i_qMin/1
  i_q/1 -> [i_q]
  [i_qLimProt] -> i_qLimProt/1
  n_max1/1 -> [n_max], Gain6/1
  Gain6/1 -> [n_min]
  [n_min] -> n_min/1
  [n_max] -> n_max/1
  n_mot/1 -> [n_mot]
  [n_limProt] -> n_limProt/1
  z_ctrlMod/1 -> [z_ctrlMod]
  Relational Operator1/1 -> Logical Operator2/1
  [z_ctrlMod] -> Relational Operator2/1, Relational Operator1/1
  Logical Operator2/1 -> If1/1
  Relational Operator2/1 -> Logical Operator2/2
  CTRL_COMM/1 -> Relational Operator1/2
  CTRL_COMM1/1 -> Relational Operator2/2
  CTRL_COMM3/1 -> Relational Operator4/2
  CTRL_COMM2/1 -> Relational Operator3/2
  Relational Operator4/1 -> Logical Operator1/2
  Logical Operator1/1 -> If2/1
  [z_ctrlMod] -> Relational Operator3/1, Relational Operator4/1
  Relational Operator3/1 -> Logical Operator1/1
  [i_qMax] -> Current_Limit_Protection/2(i_qMax)
  [i_q] -> Current_Limit_Protection/1(i_q)
  [i_qMin] -> Current_Limit_Protection/3(i_qMin)
  Current_Limit_Protection/1(i_qLimProt) -> [i_qLimProt]
  [n_max] -> Speed_Limit_Protection/2(n_max)
  [n_mot] -> Speed_Limit_Protection/1(n_mot)
  [n_min] -> Speed_Limit_Protection/3(n_min)
  Speed_Limit_Protection/1(n_limProt) -> [n_limProt]
  If1/1 -> Current_Limit_Protection/Action
  If2/1 -> Speed_Limit_Protection/Action
  i_qMax_M1/1 -> MinMax/2

== system BLDCmotorControl_FOC_R2017b_fixdt_speedDeriv/BLDC_controller/BLDC_controller/F03_Field_Oriented_Control/Open_Mode ==
  note: This will reduce the control command to 0 with a predefined rate.
  V_qPrev : Inport
  Action Port : ActionPort  InitializeStates=reset  ActionType=default
  Constant23 : Constant  Value=0  OutDataTypeStr=Inherit: Inherit via back propagation
  Data Type Conversion : DataTypeConversion  OutDataTypeStr=fixdt(1,28,16)
  Gain3 : Gain  Tag=struct('comment',struct('text','','placement',1),'logdata',struct('maxnumvals',inf,'plotchannels',[],'loggingmode',3,'channels',1),'output',struct('variable','','description','','name','$S_$B','width',1,'address','','max',NaN,'min',NaN,'class','default','type','CONTINUOUS','scaling','','lsb',1,'offset',0,'arb',0,'freeze',1,'unit','','autoscalingmode',1,'lowerheadroom',1,'upperheadroom',1,'headroomunit','bit','keepdatatype',1,'checkmin',0,'checkmax',0,'castoutput',0,'show',0),'gain',struct('variable','','description','','name','$S_$B_gain','width',1,'address','','max',NaN,'min',NaN,'class','default','type','CONTINUOUS','scaling','','lsb',1,'offset',0,'arb',0,'freeze',1,'unit','','keepdatatype',1,'value','1','scalar',0,'tolerance',1),'scalingvalid',0,'date',730486)  Gain=-1  RndMeth=Zero  OutDataTypeStr=Inherit: Same as input
  Rate_Limiter : BLDC_controller_Lib/Rate_Limiter  SystemSampleTime=-1
  dV_openRate : Constant  Value=dV_openRate  OutDataTypeStr=fixdt(1,28,16)
  for merge : Gain  Tag=struct('comment',struct('text','','placement',1),'logdata',struct('maxnumvals',inf,'plotchannels',[],'loggingmode',3,'channels',1),'output',struct('variable','','description','','name','$S_$B','width',1,'address','','max',NaN,'min',NaN,'class','default','type','CONTINUOUS','scaling','','lsb',1,'offset',0,'arb',0,'freeze',1,'unit','','autoscalingmode',1,'lowerheadroom',1,'upperheadroom',1,'headroomunit','bit','keepdatatype',1,'checkmin',0,'checkmax',0,'castoutput',0,'show',0),'gain',struct('variable','','description','','name','$S_$B_gain','width',1,'address','','max',NaN,'min',NaN,'class','default','type','CONTINUOUS','scaling','','lsb',1,'offset',0,'arb',0,'freeze',1,'unit','','keepdatatype',1,'value','1','scalar',0,'tolerance',1),'scalingvalid',0,'date',730486)  OutDataTypeStr=fixdt(1,16,4)  RndMeth=Zero
  rising_edge_init : BLDC_controller_Lib/rising_edge_init
  V_qOpen : Outport
  wires:
  V_qPrev/1 -> [V_qPrev]
  Constant23/1 -> Rate_Limiter/1
  rising_edge_init/1 -> Rate_Limiter/3
  Gain3/1 -> Rate_Limiter/5
  dV_openRate/1 -> Gain3/1, Rate_Limiter/4
  for merge/1 -> [V_qOpen]
  [V_qOpen] -> V_qOpen/1
  Rate_Limiter/1 -> for merge/1
  [V_qPrev] -> Data Type Conversion/1
  Data Type Conversion/1 -> Rate_Limiter/2

== system BLDCmotorControl_FOC_R2017b_fixdt_speedDeriv/BLDC_controller/BLDC_controller/F03_Field_Oriented_Control/Outliers_Removal_and_Filtering ==
  i_qRaw : Inport
  i_dRaw : Inport  Port=2
  i_DCLink : Inport  Port=3
  DCLink_Current_Available : Subsystem
  DCLink_Current_NOT_Available : Subsystem
  If1 : If  IfExpression=u1 ~= 0
  Merge : Merge
  Merge1 : Merge
  b_DCLinkCurrAvail : Constant  Value=b_DCLinkCurrAvail  OutDataTypeStr=boolean
  i_q : Outport
  i_d : Outport  Port=2
  wires:
  [i_d] -> i_d/1
  [i_q] -> i_q/1
  i_qRaw/1 -> [i_qRaw]
  i_dRaw/1 -> [i_dRaw]
  [i_qRaw] -> DCLink_Current_NOT_Available/1(i_qRaw)
  [i_dRaw] -> DCLink_Current_NOT_Available/2(i_dRaw)
  If1/1 -> DCLink_Current_Available/Action
  i_DCLink/1 -> [i_DCLink]
  [i_dRaw] -> DCLink_Current_Available/2(i_dRaw)
  [i_qRaw] -> DCLink_Current_Available/1(i_qRaw)
  [i_DCLink] -> DCLink_Current_Available/3(i_DCLink)
  b_DCLinkCurrAvail/1 -> If1/1
  DCLink_Current_NOT_Available/1(i_qNoDCLink) -> [i_qNoDCLink]
  DCLink_Current_NOT_Available/2(i_dNoDCLink) -> [i_dNoDCLink]
  DCLink_Current_Available/1(i_qDCLink) -> [i_qDCLink]
  DCLink_Current_Available/2(i_dDCLink) -> [i_dDCLink]
  Merge1/1 -> [i_d]
  If1/2 -> DCLink_Current_NOT_Available/Action
  [i_qNoDCLink] -> Merge/2
  [i_qDCLink] -> Merge/1
  [i_dDCLink] -> Merge1/1
  [i_dNoDCLink] -> Merge1/2
  Merge/1 -> [i_q]
